simulink model "House_Temperature"  (R2021a)
settings: Solver=VariableStepAuto  StartTime=0.0  StopTime=48  FixedStep=1  RelTol=1e-3
values from neighbouring files (symbols this model uses):
  c = 1005.4    [Model_Inputs.m]
  cost = 2.5/(3.6*10^6)    (= 6.94444444444e-07)    [Model_Inputs.m]
  M = 5987.7684    [Model_Inputs.m]
  Mdot = 3600    [Model_Inputs.m]
  Req = 0.0000004    (= 4e-07)    [Model_Inputs.m]
  Theater = 50    [Model_Inputs.m]
settings Model: Creator=gopin  LastModifiedBy=gopin

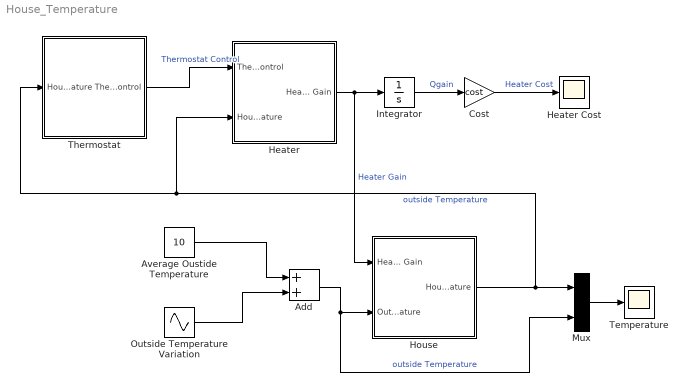
== system House_Temperature ==
  Add : Sum
  Average Oustide Temperature : Constant  Value=10
  Cost : Gain  Gain=cost
  Heater : Subsystem
      mask Display: image('D:\Decibel_Lab_BMS_Course\Course_Content\Module_3\Simulink_Practice_Project\Thermalmodelofhousepics-200527-100907\house-radiators-a-radiator-attached-to-the-wall-in-a-home-house-radiators-for-sale-near-me.jpg'); % Use "Edit Image" on toolstrip to change.
  Heater Cost : Scope
  House : Subsystem
      mask Display: image('D:\Decibel_Lab_BMS_Course\Course_Content\Module_3\Simulink_Practice_Project\Thermalmodelofhousepics-200527-100907\modern-home-exterior-gray-scheme-792ab713.jpg'); % Use "Edit Image" on toolstrip to change.
  Integrator : Integrator
  Mux : Mux  Inputs=2
  Outside Temperature Variation : Sin  Amplitude=5  Frequency=2*pi/24  SampleTime=0
  Temperature : Scope
  Thermostat : Subsystem
      mask Display: image('D:\Decibel_Lab_BMS_Course\Course_Content\Module_3\Simulink_Practice_Project\Thermalmodelofhousepics-200527-100907\Themostat.jpg'); % Use "Edit Image" on toolstrip to change.
  wires:
  Average Oustide Temperature/1 -> Add/1
  Outside Temperature Variation/1 -> Add/2
  Add/1 -> House/2(Outside Temperature), Mux/2  "outside Temperature"
  Mux/1 -> Temperature/1
  Heater/1(Heater Gain) -> House/1(Heater Gain), Integrator/1  "Heater Gain"
  Thermostat/1(Thermostat control) -> Heater/1(Thermostat Control)  "Thermostat Control"
  Integrator/1 -> Cost/1  "Qgain"
  Cost/1 -> Heater Cost/1  "Heater Cost"
  House/1(House Temperature) -> Heater/2(House Temperature), Thermostat/1(House Temperature), Mux/1  "outside Temperature"

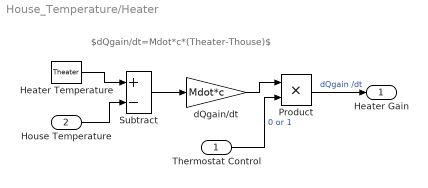
== system House_Temperature/Heater ==
  note: $dQgain/dt=Mdot*c*(Theater-Thouse)$
  Thermostat Control : Inport
  House Temperature : Inport  Port=2
  Heater Temperature : Constant  Value=Theater
  Product : Product
  Subtract : Sum  Inputs=+-
  dQgain/dt : Gain  Gain=Mdot*c
  Heater Gain : Outport
  wires:
  Heater Temperature/1 -> Subtract/1
  House Temperature/1 -> Subtract/2
  Subtract/1 -> dQgain/dt/1
  Product/1 -> Heater Gain/1  "dQgain /dt"
  dQgain/dt/1 -> Product/1
  Thermostat Control/1 -> Product/2  "0 or 1"

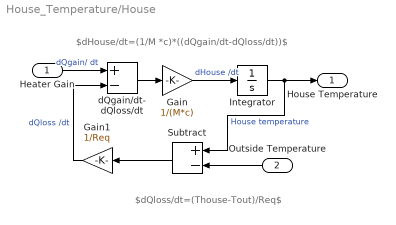
== system House_Temperature/House ==
  note: $dHouse/dt=(1/M *c)*((dQgain/dt-dQloss/dt))$
  note: $dQloss/dt=(Thouse-Tout)/Req$
  Heater Gain : Inport
  Outside Temperature : Inport  Port=2
  Gain : Gain  Gain=1/(M*c)
  Gain1 : Gain  Gain=1/Req
  Integrator : Integrator
  Subtract : Sum  Inputs=+-
  dQgain/dt- dQloss/dt : Sum  Inputs=+-
  House Temperature : Outport
  wires:
  Outside Temperature/1 -> Subtract/2
  Subtract/1 -> Gain1/1
  Integrator/1 -> Subtract/1, House Temperature/1  "House temperature"
  dQgain/dt- dQloss/dt/1 -> Gain/1
  Gain/1 -> Integrator/1  "dHouse /dt"
  Gain1/1 -> dQgain/dt- dQloss/dt/2  "dQloss /dt"
  Heater Gain/1 -> dQgain/dt- dQloss/dt/1  "dQgain/ dt"

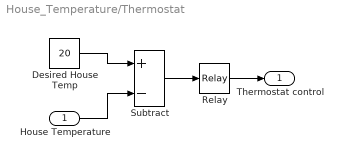
== system House_Temperature/Thermostat ==
  House Temperature : Inport
  "Desired House Temp " : Constant  Value=20
  Relay : Relay  OnSwitchValue=2  OffSwitchValue=-2
  Subtract : Sum  Inputs=+-
  Thermostat control : Outport
  wires:
  "Desired House Temp "/1 -> Subtract/1
  House Temperature/1 -> Subtract/2
  Subtract/1 -> Relay/1
  Relay/1 -> Thermostat control/1
